simulink model "pv_nmpp_2"  (R2024b)
settings: Solver=ode23tb  StartTime=0.0  StopTime=0.25  RelTol=1e-6
undefined symbols (not defined in the file): Ion, Lithium
libraries: spsDiodeLib x13, spsPVArrayLib x13, spsCurrentMeasurementLib x4, spsSeriesRLCBranchLib x4, spsVoltageMeasurementLib x4, simulink x2, spsBatteryLib x1, spsControlledVoltageSourceLib x1, spsGroundLib x1, spsMosfetLib x1, spsPWMGeneratorDCDCLib x1, spspowerguiLib x1
settings Model: Creator=vaide  LastModifiedBy=DILEEP
settings OptimizationCC: ReuseModelBlockBuffer=off
settings RTWCC: GPUComputeCapability=3.5

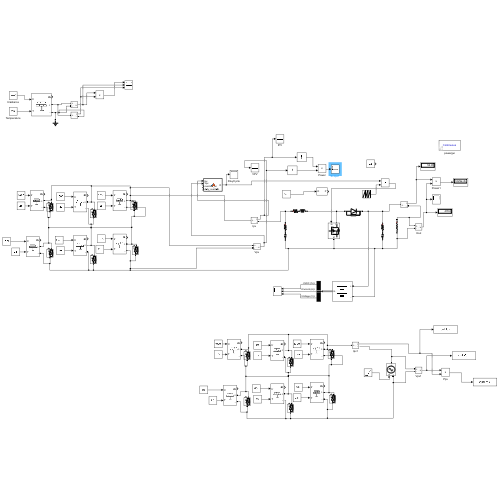
[thumbnail: Simulink's stored preview of the top-level diagram]
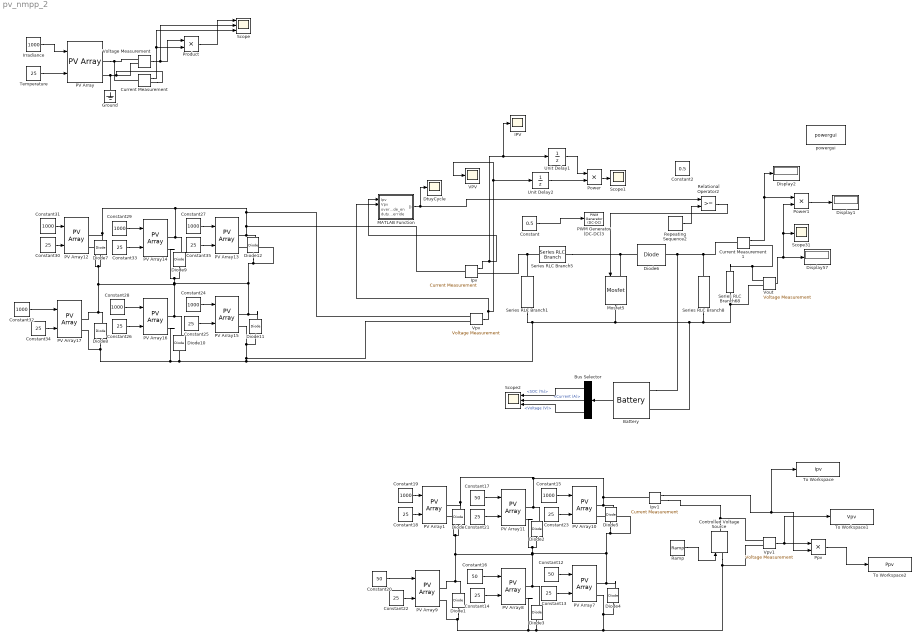
== system pv_nmpp_2 ==
  Battery : spsBatteryLib/Battery  BatType=Lithium-Ion  NomV=450  NomQ=5.4  SOC=100  Batt_Tr=30  PresetModel=off  MaxQ=5.4  MinV=337.5  FullV=523.7942  Dis_rate=2.3478  R=0.83333  Normal_OP=4.8835  expZone="[486.1736     0.2653043]"
  Bus Selector : BusSelector  OutputSignals=SOC (%),Current (A),Voltage (V)
  Constant : Constant  Value=0.5
  Constant{12,16..17,20} (4 alike) : Constant  Value=50
  Constant{13..14,18,21..23,25..26,30,33..35} (12 alike) : Constant  Value=25
  Constant{15,19,24,27..29,31..32} (8 alike) : Constant  Value=1000
  Constant2 : Constant  Value=0.5
  Controlled Voltage Source : spsControlledVoltageSourceLib/Controlled Voltage Source  Initialize=on  Source_Type=DC  Amplitude=0  Phase=0  Frequency=0  Measurements=None
  Current Measurement : spsCurrentMeasurementLib/Current Measurement  PhasorSimulation=off  OutputType=Complex  PSBequivalent=0
  Current Measurement1 : spsCurrentMeasurementLib/Current Measurement  PhasorSimulation=off  OutputType=Complex  PSBequivalent=0
  Diode{,1..5,7..12} (12 alike) : spsDiodeLib/Diode  Ron=0.001  Lon=0  Vf=0.8  IC=0  UseSnubber=0  Rs=500  Cs=250e-9  Measurements=on
  Diode6 : spsDiodeLib/Diode  Ron=1e-7  Lon=0  Vf=0  IC=0  UseSnubber=0  Rs=1e6  Cs=1e6  Measurements=off
  Display1 : Display
  Display2 : Display
  Display57 : Display
  DtuyCycle : Scope
  Ground : spsGroundLib/Ground  LConnTagsString=a
  IPV : Scope
  Ipv : spsCurrentMeasurementLib/Current Measurement  PhasorSimulation=off  OutputType=Complex  PSBequivalent=0
  Ipv1 : spsCurrentMeasurementLib/Current Measurement  PhasorSimulation=off  OutputType=Complex  PSBequivalent=0
  Irradiance : Constant  Value=1000
  MATLAB Function : MATLAB Function  TreatAsAtomicUnit=on  SystemSampleTime=1e-4
  Mosfet5 : spsMosfetLib/Mosfet  Ron=1e-7  Lon=0  Rd=1e-10  Vfd=0  IC=0  Rs=inf  Cs=0  Measurements=off
  PV Array : spsPVArrayLib/PV Array  Npar=40  Nser=10  PlotType=array @ 1000 W/m2 & specified temperatures  S_vec="[ 1000  500  100 ]"  Temp_C_vec="[ 45 25  ]"  ModuleName=User-defined  PlotWhenSelected=off  Pm=213.15  Ncell=60  Voc=36.3  Isc=7.84  Vm=29  Im=7.35  beta_Voc_pc=-0.36099  alpha_Isc_pc=0.102  beta_Voc=-0.13104  alpha_Isc=0.0079968  IL=7.8654  I0=2.9273e-10  nI=0.98119  Rsh=313.0553  Rs=0.39381  RobustModel=off  RobustCellTemperature=313.3991  BAL=on  Tc=1e-6  Tfilter=5e-5
  PV Array{1,7..17} (12 alike) : spsPVArrayLib/PV Array  Npar=1  Nser=1  PlotType=array @ 25 deg.C & specified irradiances  S_vec="[ 1000  500  100 ]"  Temp_C_vec="[ 45 25  ]"  ModuleName=Tata Power Solar Systems TP265LBZ  PlotWhenSelected=off  Pm=264.942  Ncell=72  Voc=43.7  Isc=8.01  Vm=35.9  Im=7.38  beta_Voc_pc=-0.33  alpha_Isc_pc=0.063795  beta_Voc=-0.14421  alpha_Isc=0.00511  IL=8.0299  I0=9.1111e-11  nI=0.93887  Rsh=138.0645  Rs=0.34314  RobustModel=off  RobustCellTemperature=313.3991  BAL=on  Tc=1e-6  Tfilter=5e-5
  PWM Generator (DC-DC)3 : spsPWMGeneratorDCDCLib/PWM Generator (DC-DC)  Fsw=5000  Ts=0.0001
  Power : Product
  Power1 : Product
  Ppv : Product
  Product : Product
  Ramp : simulink/Sources/Ramp  slope=43.7*2*4  start=0  InitialOutput=0
  Relational Operator2 : RelationalOperator  OutDataTypeStr=boolean  RndMeth=Simplest  InputSameDT=off
  Repeating Sequence2 : simulink/Sources/Repeating Sequence  rep_seq_t=[0 0.0002]  rep_seq_y=[0 1]
  Scope : Scope  NumInputPorts=3
  Scope1 : Scope
  Scope2 : Scope  NumInputPorts=3
  Scope31 : Scope
  Series RLC Branch1 : spsSeriesRLCBranchLib/Series RLC Branch  LConnTagsString=__new0  RConnTagsString=__new0  BranchType=RC  Resistance=0.01  Inductance=1e-3  SetiL0=off  InitialCurrent=0  Capacitance=150e-6  Setx0=on  InitialVoltage=800  Measurements=None
  Series RLC Branch5 : spsSeriesRLCBranchLib/Series RLC Branch  LConnTagsString=__new0  RConnTagsString=__new0  BranchType=RL  Resistance=0.1  Inductance=0.0003  SetiL0=off  InitialCurrent=0  Capacitance=1e-6  Setx0=off  InitialVoltage=0  Measurements=None
  Series RLC Branch68 : spsSeriesRLCBranchLib/Series RLC Branch  LConnTagsString=__new0  RConnTagsString=__new0  BranchType=R  Resistance=8.71  Inductance=1e-3  SetiL0=off  InitialCurrent=0  Capacitance=1e-6  Setx0=off  InitialVoltage=0  Measurements=None
  Series RLC Branch8 : spsSeriesRLCBranchLib/Series RLC Branch  LConnTagsString=__new0  RConnTagsString=__new0  BranchType=RC  Resistance=0.01  Inductance=1e-3  SetiL0=off  InitialCurrent=0  Capacitance=470e-6  Setx0=on  InitialVoltage=800  Measurements=None
  Temperature : Constant  Value=25
  To Workspace : ToWorkspace  VariableName=Ipv  SaveFormat=Structure With Time  SampleTime=-1
  To Workspace1 : ToWorkspace  VariableName=Vpv  SaveFormat=Structure With Time  SampleTime=-1
  To Workspace2 : ToWorkspace  VariableName=Ppv  SaveFormat=Structure With Time  SampleTime=-1
  Unit Delay1 : UnitDelay  SampleTime=1e-4  HasFrameUpgradeWarning=on
  Unit Delay2 : UnitDelay  SampleTime=1e-4  HasFrameUpgradeWarning=on
  VPV : Scope
  Voltage Measurement : spsVoltageMeasurementLib/Voltage Measurement  PhasorSimulation=off  OutputType=Complex  PSBequivalent=0
  Vout : spsVoltageMeasurementLib/Voltage Measurement  PhasorSimulation=off  OutputType=Complex  PSBequivalent=0
  Vpv : spsVoltageMeasurementLib/Voltage Measurement  PhasorSimulation=off  OutputType=Complex  PSBequivalent=0
  Vpv1 : spsVoltageMeasurementLib/Voltage Measurement  PhasorSimulation=off  OutputType=Complex  PSBequivalent=0
  powergui : spspowerguiLib/powergui  Priority=1  SimulationMode=Continuous  SampleTime=1e-5  frequency=60  Iterations=50  frequencyindice=0  Pbase=100e6  ErrMax=1e-4  UnitsV=kV  UnitsW=MW  buscounter=0  FunctionMessages=off  echomessages=off  EnableUseOfTLC=off  CurrentSourceSwitches=off  DisableSnubberDevices=off  DisableRonSwitches=off  DisableVfSwitches=off  DisplayEquations=off  AutomaticDiscreteSolvers=off  SolverType=Tustin/Backward Euler (TBE)  Interpol=off  ExternalGateDelay=off  methode=off  Ts=100  x0status=blocks  SPID=on  SwTol=0  HookPort=off  NonlinearTolerance=1e-4  nMaxIteration=100  ContinueOnMaxIteration=off  RestoreLinks=warning  ResistiveCurrentMeasurement=off  Frange=[0:2:500]  Ylog=off  Xlog=on  ShowGrid=off  save=off  variable=ZData  structure=0  ZoomFFT=off  StartTime=0.0  cycles=1  DisplayStyle=1  fundamental=60  FreqAxis=off  MaxFrequency=1000  frequencyindicesteady=1  RmsSteady=1  display=off
  wires:
  Voltage Measurement/1 -> Scope/2, Product/1
  Current Measurement/1 -> Scope/3, Product/2
  Irradiance/1 -> PV Array/1
  Temperature/1 -> PV Array/2
  Product/1 -> Scope/1
  Vout/1 -> Power1/2, Scope31/1, Display57/1
  Ipv/1 -> IPV/1, Unit Delay1/1, MATLAB Function/1(Ipv)
  Vpv/1 -> VPV/1, Unit Delay2/1, MATLAB Function/2(Vpv)
  Power/1 -> Scope1/1
  MATLAB Function/1(D) -> Relational Operator2/1, DtuyCycle/1
  Unit Delay1/1 -> Power/1
  Unit Delay2/1 -> Power/2
  Constant/1 -> PWM Generator (DC-DC)3/1
  Repeating Sequence2/1 -> Relational Operator2/2
  Relational Operator2/1 -> Mosfet5/1
  Constant17/1 -> PV Array11/1
  Constant16/1 -> PV Array8/1
  Constant12/1 -> PV Array7/1
  Constant15/1 -> PV Array10/1
  Constant19/1 -> PV Array1/1
  Constant22/1 -> PV Array9/2
  Constant23/1 -> PV Array10/2
  Constant21/1 -> PV Array11/2
  Constant13/1 -> PV Array7/2
  Constant20/1 -> PV Array9/1
  Constant14/1 -> PV Array8/2
  Constant18/1 -> PV Array1/2
  Vpv1/1 -> To Workspace1/1, Ppv/1
  Ipv1/1 -> To Workspace/1, Ppv/2
  Ppv/1 -> To Workspace2/1
  Ramp/1 -> Controlled Voltage Source/1
  Constant31/1 -> PV Array12/1
  Constant32/1 -> PV Array17/1
  Constant35/1 -> PV Array13/2
  Constant26/1 -> PV Array16/2
  Constant27/1 -> PV Array13/1
  Constant33/1 -> PV Array14/2
  Constant34/1 -> PV Array17/2
  Constant24/1 -> PV Array15/1
  Constant30/1 -> PV Array12/2
  Constant25/1 -> PV Array15/2
  Constant28/1 -> PV Array16/1
  Constant29/1 -> PV Array14/1
  Battery/1 -> Bus Selector/1
  Bus Selector/1 -> Scope2/1  "<SOC (%)>"
  Bus Selector/2 -> Scope2/2  "<Current (A)>"
  Bus Selector/3 -> Scope2/3  "<Voltage (V)>"
  Current Measurement1/1 -> Display2/1, Power1/1
  Power1/1 -> Display1/1
  connections:
  PV Array/RConn1 -- Current Measurement/LConn1 -- Voltage Measurement/LConn1
  PV Array/RConn2 -- Ground/LConn1 -- Current Measurement/RConn1 -- Voltage Measurement/LConn2
  Ipv/RConn1 -- Series RLC Branch1/LConn1 -- Series RLC Branch5/LConn1
  Diode6/LConn1 -- Series RLC Branch5/RConn1 -- Mosfet5/LConn1
  Series RLC Branch8/LConn1 -- Current Measurement1/LConn1 -- Battery/LConn1 -- Diode6/RConn1
  Ipv1/RConn1 -- Vpv1/LConn1 -- Controlled Voltage Source/RConn1
  Diode4/RConn1 -- PV Array9/RConn1 -- Diode1/RConn1 -- PV Array1/RConn2 -- Diode/LConn1 -- PV Array8/RConn1 -- Diode3/RConn1 -- PV Array11/RConn2 -- Diode2/LConn1 -- Diode5/LConn1 -- PV Array10/RConn2 -- PV Array7/RConn1
  PV Array7/RConn2 -- Vpv1/LConn2 -- Controlled Voltage Source/LConn1 -- Diode1/LConn1 -- PV Array9/RConn2 -- PV Array8/RConn2 -- Diode3/LConn1 -- Diode4/LConn1
  PV Array11/RConn1 -- Ipv1/LConn1 -- PV Array10/RConn1 -- Diode5/RConn1 -- Diode/RConn1 -- PV Array1/RConn1 -- Diode2/RConn1
  Diode11/RConn1 -- PV Array15/RConn1 -- PV Array13/RConn2 -- Diode12/LConn1 -- Diode9/LConn1 -- PV Array14/RConn2 -- Diode7/LConn1 -- PV Array12/RConn2 -- PV Array17/RConn1 -- Diode8/RConn1 -- Diode10/RConn1 -- PV Array16/RConn1
  Series RLC Branch8/RConn1 -- Vout/LConn2 -- Series RLC Branch68/RConn1 -- Battery/LConn2 -- Diode10/LConn1 -- PV Array17/RConn2 -- Diode8/LConn1 -- PV Array16/RConn2 -- Vpv/LConn2 -- PV Array15/RConn2 -- Diode11/LConn1 -- Series RLC Branch1/RConn1 -- Mosfet5/RConn1
  PV Array13/RConn1 -- Vpv/LConn1 -- PV Array12/RConn1 -- Diode7/RConn1 -- Diode9/RConn1 -- PV Array14/RConn1 -- Ipv/LConn1 -- Diode12/RConn1
  Vout/LConn1 -- Current Measurement1/RConn1 -- Series RLC Branch68/LConn1

== matlab function pv_nmpp_2/MATLAB Function ==
  data: Ipv input; D output; Vpv input; override_en input; duty_override input
function D = MPPT_TWC(Ipv, Vpv, override_en, duty_override)
%#codegen
% Modified Three-Point Weight Comparison (MTWC) MPPT
% Extended: supports duty override, stuck-detection and escape jump
% Inputs:
%  - Ipv (A), Vpv (V)
%  - override_en (0/1) : when 1, use duty_override directly (force non-MPP)
%  - duty_override (0..1) : forced duty when override_en==1
% Output:
%  - D : duty cycle (0..1)

%% --- Tunable Parameters ---
Vmax    = 35;       % expected PV MPP voltage (V) - tune for your panel
Dmin    = 0.002;    % min step
DmMax   = 0.05;     % max step
k       = 5;        % exponential slope for Dm
Di0     = 0.5;      % initial duty
% stuck/escape parameters
N_no_improve = 80;      % number of samples without improvement before escape
escape_step   = 0.18;   % magnitude of escape jump (fraction of duty)
Tscan_samples = 1200;   % periodic scan interval in samples (optional)
seedRand = 12345;       % random seed for reproducibility (only init)

%% --- Persistent states ---
persistent P1i P2i Di Ki V_old initFlag bestP samples_no_improve sample_count rngState

if isempty(initFlag)
    P1i = 1e-6; P2i = 1e-6;
    Di = Di0; Ki = 1; V_old = 0;
    bestP = 0;
    samples_no_improve = 0;
    sample_count = 0;
    rngState = seedRand;
    initFlag = true;
end

%% Defensive input checks
if isnan(Ipv) || isnan(Vpv) || isinf(Ipv) || isinf(Vpv)
    D = Di;
    return;
end

%% Instantaneous power (non-negative)
P_now = Vpv * Ipv;
if P_now < 0
    P_now = 0;
end

%% Adaptive step size Dm (same idea as your original)
if Vmax <= 0
    Dm = max(Dmin, min(DmMax, 0.01));
else
    rel_err = abs(Vpv - Vmax) / max(1e-6, Vmax);
    Dm = Dmin + (DmMax - Dmin) * (1 - exp(-k * rel_err));
end
Dm = min(max(Dm, Dmin), DmMax);

%% If override enabled -> force duty (useful to create non-MPP)
if nargin >= 3 && override_en == 1
    % forced duty (immediately)
    Di = min(max(duty_override, 0), 1);
    % update memories but do not change search behaviour
    P2i = P1i; P1i = P_now; V_old = Vpv;
    D = Di;
    return;
end

%% --- Original Three-point weight comparisons (kept) ---
PA = P_now; PB = P1i; PC = P2i;
M = 0;
if PB >= PA
    M = M + 1;
else
    M = M - 1;
end
if PA > PC
    M = M + 1;
else
    M = M - 1;
end

K = Ki;
if M == 2
    if Ki == 1
        Di = Di + Dm; K = 1;
    else
        Di = Di + 3*Dm; K = 1;
    end
elseif M == -2
    if Ki == -1
        Di = Di - Dm; K = -1;
    else
        Di = Di - 3*Dm; K = -1;
    end
else
    if PB >= PA && PA <= PC
        K = 0; % near MPP
    else
        if Vpv < V_old
            Di = Di + Dm; K = 1;
        else
            Di = Di - Dm; K = -1;
        end
    end
end

%% Clamp
Di = min(max(Di, 0), 1);

%% --- Update Ki memory ---
if K ~= 0
    Ki = K;
end

%% --- Stuck detection & escape logic ---
% update sample counters and bestP
sample_count = sample_count + 1;
if P_now > bestP + 1e-6  % improvement (tiny tolerance)
    bestP = P_now;
    samples_no_improve = 0;
else
    samples_no_improve = samples_no_improve + 1;
end

% if stuck for too long, apply an escape action (large random jump)
if samples_no_improve >= N_no_improve
    % reproducible random jitter: linear congruential simple RNG
    rngState = mod(1664525 * rngState + 1013904223, 2^32);
    r = double(mod(rngState,1000))/1000 - 0.5; % range -0.5..0.5
    % make a jump proportional to escape_step and sign of r
    jump = sign(r) * escape_step;
    Di = Di + jump;
    % clamp and reset stuck counter and bestP (so we can detect improvement)
    Di = min(max(Di,0),1);
    samples_no_improve = 0;
    bestP = P_now;
end

% optional periodic coarse scan: every Tscan_samples do a moderate jump
if sample_count >= Tscan_samples
    Di = Di + 0.5 * escape_step;          % moderate deterministic jump
    Di = min(max(Di,0),1);
    sample_count = 0;
    bestP = P_now;
    samples_no_improve = 0;
end

%% Update stored power history and previous voltage
P2i = P1i;
P1i = P_now;
V_old = Vpv;

%% Output
D = Di;

end
